simulink model "sistema_furuta"  (R2024a)
settings: Solver=VariableStepAuto  StartTime=0.0  StopTime=0.5  RelTol=1e-3
settings Model: Creator=PC  LastModifiedBy=PC
settings SolverCC: MaxConsecutiveMinStep=100
settings RTWCC: GPUComputeCapability=3.5

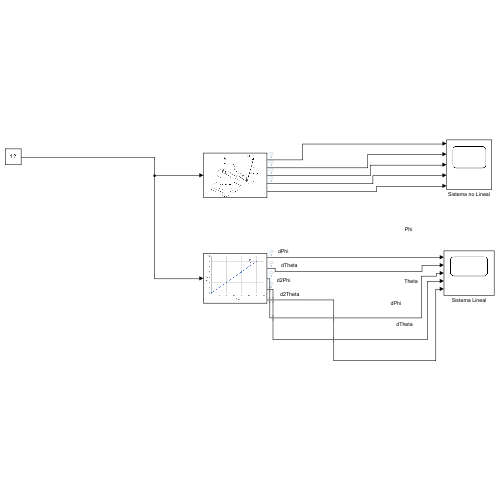
[thumbnail: Simulink's stored preview of the top-level diagram]
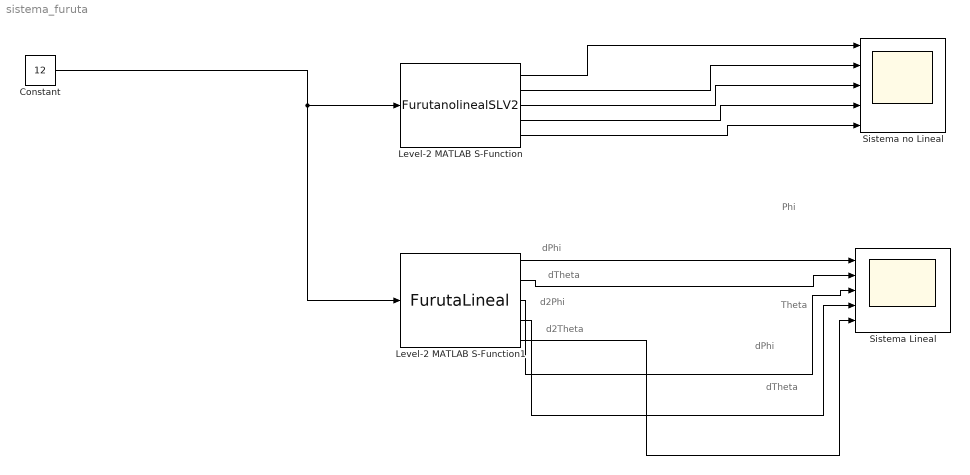
== system sistema_furuta ==
  note: dTheta
  note: dPhi
  note: Theta
  note: Phi
  note: d2Theta
  note: d2Phi
  note: dTheta
  note: dPhi
  Constant : Constant  Value=12
  Level-2 MATLAB S-Function : M-S-Function  FunctionName=FurutanolinealSLV2  mask{Xi=0, g=0, J=0, M_2=0, l_bi=0, C_x=0, C_z=0, I_x=0, I_z=0}
      mask prompts: Xi "Parametros iniciales (Xi)"
      mask Display: image('mascara2.png');
  Level-2 MATLAB S-Function1 : M-S-Function  FunctionName=FurutaLineal  mask{Xi=0, g=0, J=0, M_2=0, l_bi=0, C_x=0, C_z=0, I_x=0, I_z=0}
      mask prompts: Xi "Parametros iniciales (Xi)"
      mask Display: image('Lineal.png');
  Sistema Lineal : Scope  NumInputPorts=5
  Sistema no Lineal : Scope  NumInputPorts=5
  wires:
  Constant/1 -> Level-2 MATLAB S-Function1/1, Level-2 MATLAB S-Function/1
  Level-2 MATLAB S-Function1/1 -> Sistema Lineal/1
  Level-2 MATLAB S-Function1/3 -> Sistema Lineal/3
  Level-2 MATLAB S-Function1/4 -> Sistema Lineal/4
  Level-2 MATLAB S-Function/1 -> Sistema no Lineal/1
  Level-2 MATLAB S-Function/2 -> Sistema no Lineal/2
  Level-2 MATLAB S-Function/3 -> Sistema no Lineal/3
  Level-2 MATLAB S-Function/4 -> Sistema no Lineal/4
  Level-2 MATLAB S-Function/5 -> Sistema no Lineal/5
  Level-2 MATLAB S-Function1/5 -> Sistema Lineal/5
  Level-2 MATLAB S-Function1/2 -> Sistema Lineal/2
